simulink model "Quadcopter_State_model_Arduino"  (R2023b)
settings: Solver=VariableStepAuto  StartTime=0.0  StopTime=inf  FixedStep=0.00001  MinStep=0.001  RelTol=1e-3
model workspace (MAT data in the model file):
  DesiredPitchRoll : sugfis (value not decoded)
  DesiredThrust : sugfis (value not decoded)
  DesiredYaw : sugfis (value not decoded)
  Desired_Pitch = 0
  Desired_Roll = 0
  Desired_Yaw = 0
  Desired_Z_Velocity = -3
  FuzzyMotorspeed : sugfis (value not decoded)
values from neighbouring files (symbols this model uses):
  g = 9.81    [Quadcopter_Constants.m]
  Ixx = 0.0294838    [Quadcopter_Constants.m]
  Iyy = 0.0294838    [Quadcopter_Constants.m]
  Izz = 0.058967624    [Quadcopter_Constants.m]
  Jr = (6e-5)*1.358    (= 8.148e-05)    [Quadcopter_Constants.m]
  kd = 1    [Quadcopter_Constants.m]
  kd_phi = 1    [Quadcopter_Constants.m]
  kd_theta = 1    [Quadcopter_Constants.m]
  kf = 1    [Quadcopter_Constants.m]
  ki = 1    [Quadcopter_Constants.m]
  ki_phi = 1    [Quadcopter_Constants.m]
  ki_theta = 1    [Quadcopter_Constants.m]
  km = 4.74157e-9    (= 4.74157e-09)    [Quadcopter_Constants.m]
  kp = 1    [Quadcopter_Constants.m]
  kp_phi = 1    [Quadcopter_Constants.m]
  kp_theta = 1    [Quadcopter_Constants.m]
  kr = (0.1)*1.358    (= 0.1358)    [Quadcopter_Constants.m]
  kt = (0.1)*1.358    (= 0.1358)    [Quadcopter_Constants.m]
  l = 0.254    [Quadcopter_Constants.m]
  m = 0.914    [Quadcopter_Constants.m]
  sample_freq = 1000    [Quadcopter_Constants.m]
undefined symbols (not defined in the file or in its folder): LF
libraries: fuzblock x18, instrumentseriallib x12, simulink_extras x6, vrlib x4, instrumentlib x3, etargetslib x1, slpidlib x1, simulink x1
(part 5 of 5)

== system Quadcopter_State_model_Arduino/PID Simulation/Sensors/Sampling ==
  X_State : Inport
  Memory : Memory
  Square Wave Generator Enable : SignalGenerator  WaveForm=square  Frequency=sample_freq  Units=rad/sec
  Switch : Switch  Criteria=u2 > Threshold  SaturateOnIntegerOverflow=off  InputSameDT=off
  X_State Sensor : Outport
  wires:
  Switch/1 -> Memory/1
  Memory/1 -> X_State Sensor/1, Switch/3
  Square Wave Generator Enable/1 -> Switch/2
  X_State/1 -> Switch/1

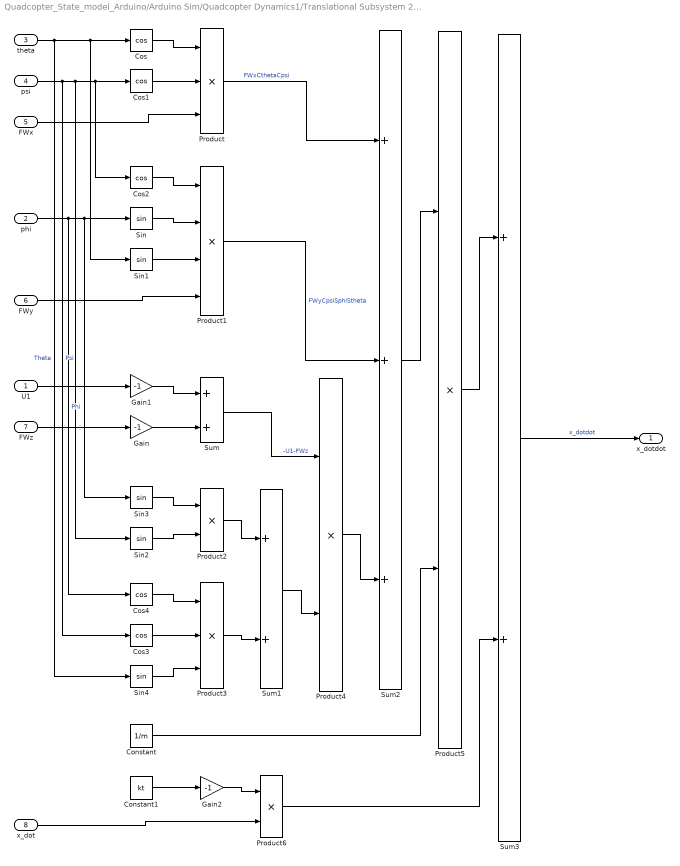
== system Quadcopter_State_model_Arduino/Arduino Sim/Quadcopter Dynamics1/Translational Subsystem 2.0/x_dotdot ==
  U1 : Inport
  phi : Inport  Port=2
  theta : Inport  Port=3
  psi : Inport  Port=4
  FWx : Inport  Port=5
  FWy : Inport  Port=6
  FWz : Inport  Port=7
  x_dot : Inport  Port=8
  Constant : Constant  Value=1/m
  Constant1 : Constant  Value=kt
  Cos{,1..4} (5 alike) : Trigonometry  Operator=cos
  Gain : Gain  Gain=-1
  Gain1 : Gain  Gain=-1
  Gain2 : Gain  Gain=-1
  Product : Product  Inputs=3
  Product1 : Product  Inputs=4
  Product{2,4..6} (4 alike) : Product
  Product3 : Product  Inputs=3
  Sin{,1..4} (5 alike) : Trigonometry
  Sum : Sum
  Sum1 : Sum
  Sum2 : Sum  Inputs=+++
  Sum3 : Sum
  x_dotdot : Outport
  wires:
  FWy/1 -> Product1/4
  x_dot/1 -> Product6/2
  U1/1 -> Gain1/1
  phi/1 -> Cos4/1, Sin3/1, Sin/1  "Phi"
  Cos1/1 -> Product/2
  FWx/1 -> Product/3
  psi/1 -> Cos3/1, Sin2/1, Cos2/1, Cos1/1  "Psi"
  Cos3/1 -> Product3/2
  Cos4/1 -> Product3/1
  Sin/1 -> Product1/2
  Product2/1 -> Sum1/1
  Gain1/1 -> Sum/1
  Sin4/1 -> Product3/3
  Product/1 -> Sum2/1  "FWxCthetaCpsi"
  Constant1/1 -> Gain2/1
  Product6/1 -> Sum3/2
  Sum3/1 -> x_dotdot/1  "x_dotdot"
  Cos/1 -> Product/1
  Gain2/1 -> Product6/1
  Constant/1 -> Product5/2
  Sin2/1 -> Product2/2
  Gain/1 -> Sum/2
  Product3/1 -> Sum1/2
  Sin3/1 -> Product2/1
  Product1/1 -> Sum2/2  "FWyCpsiSphiStheta"
  theta/1 -> Sin4/1, Sin1/1, Cos/1  "Theta"
  Sum2/1 -> Product5/1
  Sin1/1 -> Product1/3
  Cos2/1 -> Product1/1
  Product5/1 -> Sum3/1
  Sum/1 -> Product4/1  "-U1-FWz"
  FWz/1 -> Gain/1
  Sum1/1 -> Product4/2
  Product4/1 -> Sum2/3

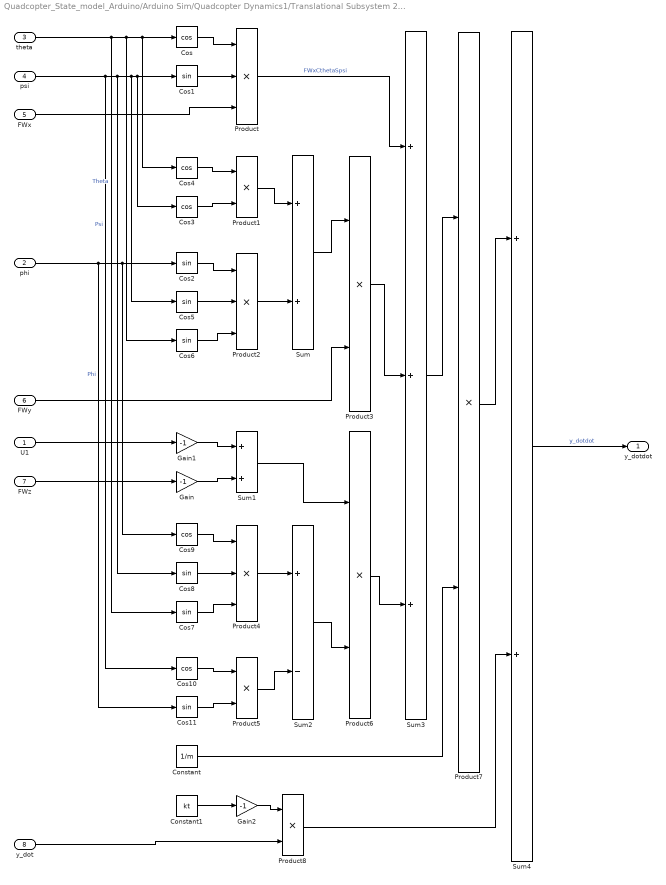
== system Quadcopter_State_model_Arduino/Arduino Sim/Quadcopter Dynamics1/Translational Subsystem 2.0/y_dotdot ==
  U1 : Inport
  phi : Inport  Port=2
  theta : Inport  Port=3
  psi : Inport  Port=4
  FWx : Inport  Port=5
  FWy : Inport  Port=6
  FWz : Inport  Port=7
  y_dot : Inport  Port=8
  Constant : Constant  Value=1/m
  Constant1 : Constant  Value=kt
  Cos{,3..4,9..10} (5 alike) : Trigonometry  Operator=cos
  Cos{1..2,5..8,11} (7 alike) : Trigonometry
  Gain : Gain  Gain=-1
  Gain1 : Gain  Gain=-1
  Gain2 : Gain  Gain=-1
  Product : Product  Inputs=3
  Product{1,3,5..8} (6 alike) : Product
  Product2 : Product  Inputs=3
  Product4 : Product  Inputs=3
  Sum : Sum
  Sum1 : Sum
  Sum2 : Sum  Inputs=+-
  Sum3 : Sum  Inputs=+++
  Sum4 : Sum
  y_dotdot : Outport
  wires:
  Product8/1 -> Sum4/2
  Product4/1 -> Sum2/1
  Gain/1 -> Sum1/2
  Sum2/1 -> Product6/2
  Product2/1 -> Sum/2
  Constant1/1 -> Gain2/1
  Cos2/1 -> Product2/1
  theta/1 -> Cos7/1, Cos6/1, Cos4/1, Cos/1  "Theta"
  psi/1 -> Cos10/1, Cos8/1, Cos5/1, Cos3/1, Cos1/1  "Psi"
  phi/1 -> Cos11/1, Cos9/1, Cos2/1  "Phi"
  Cos8/1 -> Product4/2
  Cos10/1 -> Product5/1
  y_dot/1 -> Product8/2
  FWy/1 -> Product3/2
  Cos1/1 -> Product/2
  Sum/1 -> Product3/1
  Cos5/1 -> Product2/2
  Gain2/1 -> Product8/1
  Sum4/1 -> y_dotdot/1  "y_dotdot"
  Product5/1 -> Sum2/2
  Cos3/1 -> Product1/2
  Product7/1 -> Sum4/1
  Gain1/1 -> Sum1/1
  FWx/1 -> Product/3
  Sum1/1 -> Product6/1
  Product3/1 -> Sum3/2
  Product6/1 -> Sum3/3
  Sum3/1 -> Product7/1
  Cos/1 -> Product/1
  Product/1 -> Sum3/1  "FWxCthetaSpsi"
  Cos6/1 -> Product2/3
  Cos7/1 -> Product4/3
  Cos4/1 -> Product1/1
  Cos9/1 -> Product4/1
  Cos11/1 -> Product5/2
  Product1/1 -> Sum/1
  U1/1 -> Gain1/1
  FWz/1 -> Gain/1
  Constant/1 -> Product7/2

== system Quadcopter_State_model_Arduino/Arduino Sim/Quadcopter Dynamics1/Translational Subsystem 2.0/z_dodot ==
  U1 : Inport
  phi : Inport  Port=2
  theta : Inport  Port=3
  FWx : Inport  Port=4
  FWy : Inport  Port=5
  FWz : Inport  Port=6
  z_dot : Inport  Port=7
  Constant : Constant  Value=kt
  Constant1 : Constant  Value=g
  Cos2 : Trigonometry  Operator=cos
  Cos3 : Trigonometry
  Cos4 : Trigonometry
  Cos5 : Trigonometry  Operator=cos
  Cos6 : Trigonometry  Operator=cos
  Gain{,1..2,4} (4 alike) : Gain  Gain=-1
  Gain3 : Gain  Gain=1/m
  Product : Product
  Product1 : Product  Inputs=3
  Product2 : Product  Inputs=3
  Product3 : Product
  Sum : Sum
  Sum1 : Sum  Inputs=+++
  Sum2 : Sum  Inputs=+++
  z_dotdot : Outport
  wires:
  Product3/1 -> Sum2/3
  FWy/1 -> Product1/3
  theta/1 -> Cos6/1, Cos2/1, Cos3/1  "Theta"
  z_dot/1 -> Product3/2
  phi/1 -> Cos5/1, Cos4/1  "Phi"
  Cos5/1 -> Product2/2
  Product1/1 -> Sum1/2
  Product2/1 -> Sum1/3
  Cos4/1 -> Product1/2
  U1/1 -> Gain/1
  Gain/1 -> Sum/1
  Cos2/1 -> Product1/1
  Sum/1 -> Product2/1
  Cos3/1 -> Product/2
  Gain3/1 -> Sum2/2
  Gain2/1 -> Product3/1
  FWx/1 -> Gain4/1
  Sum1/1 -> Gain3/1
  FWz/1 -> Gain1/1
  Constant/1 -> Gain2/1
  Cos6/1 -> Product2/3
  Product/1 -> Sum1/1
  Gain1/1 -> Sum/2
  Constant1/1 -> Sum2/1
  Sum2/1 -> z_dotdot/1  "z_dotdot"
  Gain4/1 -> Product/1

== system Quadcopter_State_model_Arduino/Arduino Sim/Quadcopter Dynamics1/Translational Wind Engine/Projected Areas ==
  theta : Inport
  psi : Inport  Port=2
  phi : Inport  Port=3
  Abs{,1..5} (6 alike) : Abs  SaturateOnIntegerOverflow=off
  Product{,1..5} (6 alike) : Product
  Sin{,1,4..5,8..9} (6 alike) : Trigonometry
  Sin{2..3,6..7,10..11} (6 alike) : Trigonometry  Operator=cos
  Sum : Sum
  Sum1 : Sum
  Sum2 : Sum
  Ax : Outport
  Ay : Outport  Port=2
  Az : Outport  Port=3
  wires:
  theta/1 -> Sin10/1, Sin8/1, Sin2/1, Sin/1  "theta"
  Sin6/1 -> Product3/1
  Sin9/1 -> Product4/2
  Product2/1 -> Abs2/1
  Abs2/1 -> Sum1/1
  Abs3/1 -> Sum1/2
  Sin1/1 -> Product/2
  Sin8/1 -> Product4/1
  Sin10/1 -> Product5/1
  Sin7/1 -> Product3/2
  Sin4/1 -> Product2/1
  Sin5/1 -> Product2/2
  Sin/1 -> Product/1
  Product3/1 -> Abs3/1
  Sum/1 -> Ax/1  "Ax"
  Product/1 -> Abs/1
  Product5/1 -> Abs5/1
  psi/1 -> Sin7/1, Sin5/1, Sin3/1, Sin1/1  "psi"
  Sin11/1 -> Product5/2
  Product1/1 -> Abs1/1
  Abs5/1 -> Sum2/2
  Abs4/1 -> Sum2/1
  Product4/1 -> Abs4/1
  Abs1/1 -> Sum/2
  Sin2/1 -> Product1/1
  Abs/1 -> Sum/1
  Sin3/1 -> Product1/2
  Sum1/1 -> Ay/1  "Ay"
  Sum2/1 -> Az/1  "Az"
  phi/1 -> Sin11/1, Sin9/1, Sin6/1, Sin4/1  "phi"

== system Quadcopter_State_model_Arduino/Arduino Sim/Quadcopter Dynamics1/Translational Wind Engine/Wind Forces ==
  Ax : Inport
  Ay : Inport  Port=2
  Az : Inport  Port=3
  VWx : Inport  Port=4
  VWy : Inport  Port=5
  VWz : Inport  Port=6
  Constant : Constant  Value=0.613
  Constant1 : Constant  Value=0.613
  Constant2 : Constant  Value=kt
  Constant3 : Constant  Value=kt
  Constant4 : Constant  Value=0.613
  Constant5 : Constant  Value=kt
  Product : Product  Inputs=4
  Product1 : Product  Inputs=4
  Product2 : Product  Inputs=4
  Square : Math  Operator=square
  Square1 : Math  Operator=square
  Square2 : Math  Operator=square
  FWx : Outport
  FWy : Outport  Port=2
  FWz : Outport  Port=3
  wires:
  VWz/1 -> Square2/1
  Constant4/1 -> Product2/1
  Square2/1 -> Product2/4
  Constant2/1 -> Product/3
  Ax/1 -> Product/2
  Constant5/1 -> Product2/3
  Square/1 -> Product/4
  Az/1 -> Product2/2
  Constant/1 -> Product/1
  VWx/1 -> Square/1
  Constant3/1 -> Product1/3
  VWy/1 -> Square1/1
  Square1/1 -> Product1/4
  Ay/1 -> Product1/2
  Product2/1 -> FWz/1  "FWz"
  Constant1/1 -> Product1/1
  Product/1 -> FWx/1  "FWx"
  Product1/1 -> FWy/1  "FWy"

== system Quadcopter_State_model_Arduino/Arduino Sim/Quadcopter Dynamics1/Translational Wind Engine/Wind Generation ==
  Constant1 : Constant  Value=0
  Constant3 : Constant  Value=0
  Constant5 : Constant  Value=0
  Enable Wind X : Constant  Value=0
  Enable Wind Y : Constant  Value=0
  Enable Wind Z : Constant  Value=0
  Random Number : RandomNumber  SampleTime=0.1
  Random Number1 : RandomNumber  SampleTime=0.1
  Random Number2 : RandomNumber  SampleTime=0.1
  Switch : Switch  Criteria=u2 > Threshold  SaturateOnIntegerOverflow=off  InputSameDT=off
  Switch1 : Switch  Criteria=u2 > Threshold  SaturateOnIntegerOverflow=off  InputSameDT=off
  Switch2 : Switch  Criteria=u2 > Threshold  SaturateOnIntegerOverflow=off  InputSameDT=off
  VWx : Outport
  VWy : Outport  Port=2
  VWz : Outport  Port=3
  wires:
  Random Number/1 -> Switch/1  "X wind"
  Constant3/1 -> Switch/3
  Enable Wind X/1 -> Switch/2  "Enable"
  Switch/1 -> VWx/1
  Constant1/1 -> Switch1/3
  Enable Wind Y/1 -> Switch1/2  "Enable"
  Random Number1/1 -> Switch1/1  "Y wind"
  Constant5/1 -> Switch2/3
  Enable Wind Z/1 -> Switch2/2  "Enable"
  Random Number2/1 -> Switch2/1  "Z wind"
  Switch2/1 -> VWz/1
  Switch1/1 -> VWy/1

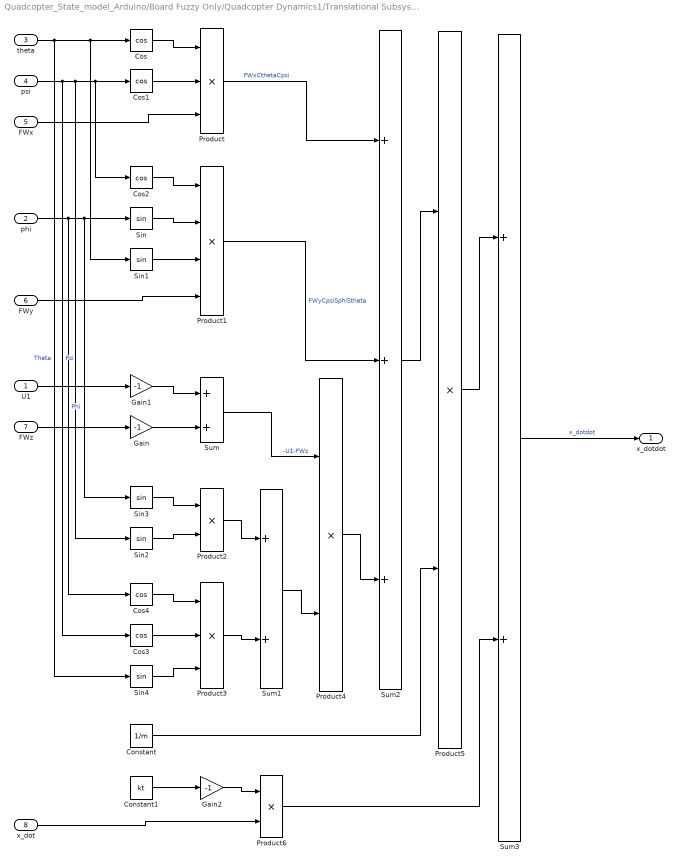
== system Quadcopter_State_model_Arduino/Board Fuzzy Only/Quadcopter Dynamics1/Translational Subsystem 2.0/x_dotdot ==
  U1 : Inport
  phi : Inport  Port=2
  theta : Inport  Port=3
  psi : Inport  Port=4
  FWx : Inport  Port=5
  FWy : Inport  Port=6
  FWz : Inport  Port=7
  x_dot : Inport  Port=8
  Constant : Constant  Value=1/m
  Constant1 : Constant  Value=kt
  Cos{,1..4} (5 alike) : Trigonometry  Operator=cos
  Gain : Gain  Gain=-1
  Gain1 : Gain  Gain=-1
  Gain2 : Gain  Gain=-1
  Product : Product  Inputs=3
  Product1 : Product  Inputs=4
  Product{2,4..6} (4 alike) : Product
  Product3 : Product  Inputs=3
  Sin{,1..4} (5 alike) : Trigonometry
  Sum : Sum
  Sum1 : Sum
  Sum2 : Sum  Inputs=+++
  Sum3 : Sum
  x_dotdot : Outport
  wires:
  FWy/1 -> Product1/4
  x_dot/1 -> Product6/2
  U1/1 -> Gain1/1
  phi/1 -> Cos4/1, Sin3/1, Sin/1  "Phi"
  Cos1/1 -> Product/2
  FWx/1 -> Product/3
  psi/1 -> Cos3/1, Sin2/1, Cos2/1, Cos1/1  "Psi"
  Cos3/1 -> Product3/2
  Cos4/1 -> Product3/1
  Sin/1 -> Product1/2
  Product2/1 -> Sum1/1
  Gain1/1 -> Sum/1
  Sin4/1 -> Product3/3
  Product/1 -> Sum2/1  "FWxCthetaCpsi"
  Constant1/1 -> Gain2/1
  Product6/1 -> Sum3/2
  Sum3/1 -> x_dotdot/1  "x_dotdot"
  Cos/1 -> Product/1
  Gain2/1 -> Product6/1
  Constant/1 -> Product5/2
  Sin2/1 -> Product2/2
  Gain/1 -> Sum/2
  Product3/1 -> Sum1/2
  Sin3/1 -> Product2/1
  Product1/1 -> Sum2/2  "FWyCpsiSphiStheta"
  theta/1 -> Sin4/1, Sin1/1, Cos/1  "Theta"
  Sum2/1 -> Product5/1
  Sin1/1 -> Product1/3
  Cos2/1 -> Product1/1
  Product5/1 -> Sum3/1
  Sum/1 -> Product4/1  "-U1-FWz"
  FWz/1 -> Gain/1
  Sum1/1 -> Product4/2
  Product4/1 -> Sum2/3

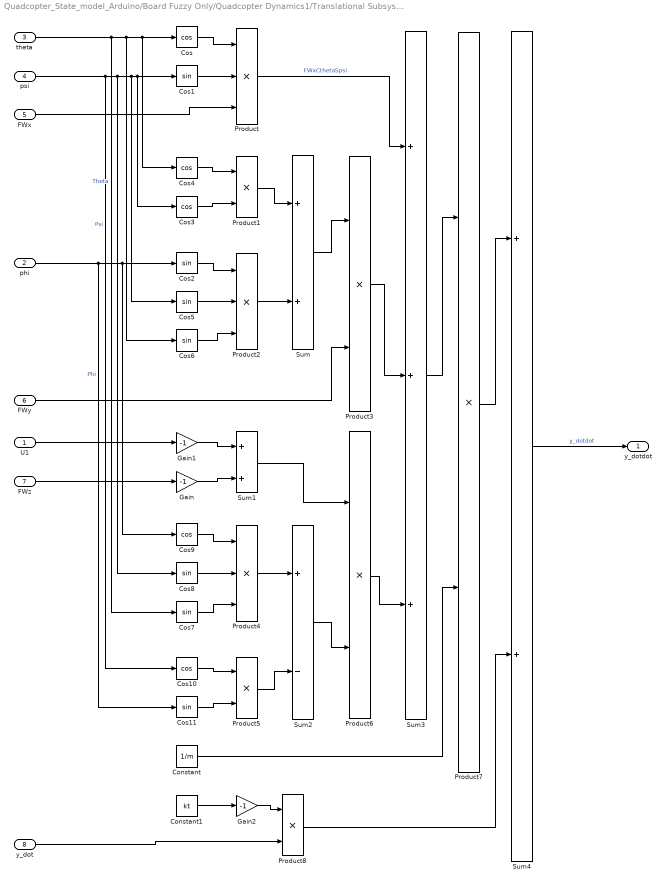
== system Quadcopter_State_model_Arduino/Board Fuzzy Only/Quadcopter Dynamics1/Translational Subsystem 2.0/y_dotdot ==
  U1 : Inport
  phi : Inport  Port=2
  theta : Inport  Port=3
  psi : Inport  Port=4
  FWx : Inport  Port=5
  FWy : Inport  Port=6
  FWz : Inport  Port=7
  y_dot : Inport  Port=8
  Constant : Constant  Value=1/m
  Constant1 : Constant  Value=kt
  Cos{,3..4,9..10} (5 alike) : Trigonometry  Operator=cos
  Cos{1..2,5..8,11} (7 alike) : Trigonometry
  Gain : Gain  Gain=-1
  Gain1 : Gain  Gain=-1
  Gain2 : Gain  Gain=-1
  Product : Product  Inputs=3
  Product{1,3,5..8} (6 alike) : Product
  Product2 : Product  Inputs=3
  Product4 : Product  Inputs=3
  Sum : Sum
  Sum1 : Sum
  Sum2 : Sum  Inputs=+-
  Sum3 : Sum  Inputs=+++
  Sum4 : Sum
  y_dotdot : Outport
  wires:
  Product8/1 -> Sum4/2
  Product4/1 -> Sum2/1
  Gain/1 -> Sum1/2
  Sum2/1 -> Product6/2
  Product2/1 -> Sum/2
  Constant1/1 -> Gain2/1
  Cos2/1 -> Product2/1
  theta/1 -> Cos7/1, Cos6/1, Cos4/1, Cos/1  "Theta"
  psi/1 -> Cos10/1, Cos8/1, Cos5/1, Cos3/1, Cos1/1  "Psi"
  phi/1 -> Cos11/1, Cos9/1, Cos2/1  "Phi"
  Cos8/1 -> Product4/2
  Cos10/1 -> Product5/1
  y_dot/1 -> Product8/2
  FWy/1 -> Product3/2
  Cos1/1 -> Product/2
  Sum/1 -> Product3/1
  Cos5/1 -> Product2/2
  Gain2/1 -> Product8/1
  Sum4/1 -> y_dotdot/1  "y_dotdot"
  Product5/1 -> Sum2/2
  Cos3/1 -> Product1/2
  Product7/1 -> Sum4/1
  Gain1/1 -> Sum1/1
  FWx/1 -> Product/3
  Sum1/1 -> Product6/1
  Product3/1 -> Sum3/2
  Product6/1 -> Sum3/3
  Sum3/1 -> Product7/1
  Cos/1 -> Product/1
  Product/1 -> Sum3/1  "FWxCthetaSpsi"
  Cos6/1 -> Product2/3
  Cos7/1 -> Product4/3
  Cos4/1 -> Product1/1
  Cos9/1 -> Product4/1
  Cos11/1 -> Product5/2
  Product1/1 -> Sum/1
  U1/1 -> Gain1/1
  FWz/1 -> Gain/1
  Constant/1 -> Product7/2

== system Quadcopter_State_model_Arduino/Board Fuzzy Only/Quadcopter Dynamics1/Translational Subsystem 2.0/z_dodot ==
  U1 : Inport
  phi : Inport  Port=2
  theta : Inport  Port=3
  FWx : Inport  Port=4
  FWy : Inport  Port=5
  FWz : Inport  Port=6
  z_dot : Inport  Port=7
  Constant : Constant  Value=kt
  Constant1 : Constant  Value=g
  Cos2 : Trigonometry  Operator=cos
  Cos3 : Trigonometry
  Cos4 : Trigonometry
  Cos5 : Trigonometry  Operator=cos
  Cos6 : Trigonometry  Operator=cos
  Gain{,1..2,4} (4 alike) : Gain  Gain=-1
  Gain3 : Gain  Gain=1/m
  Product : Product
  Product1 : Product  Inputs=3
  Product2 : Product  Inputs=3
  Product3 : Product
  Sum : Sum
  Sum1 : Sum  Inputs=+++
  Sum2 : Sum  Inputs=+++
  z_dotdot : Outport
  wires:
  Product3/1 -> Sum2/3
  FWy/1 -> Product1/3
  theta/1 -> Cos6/1, Cos2/1, Cos3/1  "Theta"
  z_dot/1 -> Product3/2
  phi/1 -> Cos5/1, Cos4/1  "Phi"
  Cos5/1 -> Product2/2
  Product1/1 -> Sum1/2
  Product2/1 -> Sum1/3
  Cos4/1 -> Product1/2
  U1/1 -> Gain/1
  Gain/1 -> Sum/1
  Cos2/1 -> Product1/1
  Sum/1 -> Product2/1
  Cos3/1 -> Product/2
  Gain3/1 -> Sum2/2
  Gain2/1 -> Product3/1
  FWx/1 -> Gain4/1
  Sum1/1 -> Gain3/1
  FWz/1 -> Gain1/1
  Constant/1 -> Gain2/1
  Cos6/1 -> Product2/3
  Product/1 -> Sum1/1
  Gain1/1 -> Sum/2
  Constant1/1 -> Sum2/1
  Sum2/1 -> z_dotdot/1  "z_dotdot"
  Gain4/1 -> Product/1

== system Quadcopter_State_model_Arduino/Board Fuzzy Only/Quadcopter Dynamics1/Translational Wind Engine/Projected Areas ==
  theta : Inport
  psi : Inport  Port=2
  phi : Inport  Port=3
  Abs{,1..5} (6 alike) : Abs  SaturateOnIntegerOverflow=off
  Product{,1..5} (6 alike) : Product
  Sin{,1,4..5,8..9} (6 alike) : Trigonometry
  Sin{2..3,6..7,10..11} (6 alike) : Trigonometry  Operator=cos
  Sum : Sum
  Sum1 : Sum
  Sum2 : Sum
  Ax : Outport
  Ay : Outport  Port=2
  Az : Outport  Port=3
  wires:
  theta/1 -> Sin10/1, Sin8/1, Sin2/1, Sin/1  "theta"
  Sin6/1 -> Product3/1
  Sin9/1 -> Product4/2
  Product2/1 -> Abs2/1
  Abs2/1 -> Sum1/1
  Abs3/1 -> Sum1/2
  Sin1/1 -> Product/2
  Sin8/1 -> Product4/1
  Sin10/1 -> Product5/1
  Sin7/1 -> Product3/2
  Sin4/1 -> Product2/1
  Sin5/1 -> Product2/2
  Sin/1 -> Product/1
  Product3/1 -> Abs3/1
  Sum/1 -> Ax/1  "Ax"
  Product/1 -> Abs/1
  Product5/1 -> Abs5/1
  psi/1 -> Sin7/1, Sin5/1, Sin3/1, Sin1/1  "psi"
  Sin11/1 -> Product5/2
  Product1/1 -> Abs1/1
  Abs5/1 -> Sum2/2
  Abs4/1 -> Sum2/1
  Product4/1 -> Abs4/1
  Abs1/1 -> Sum/2
  Sin2/1 -> Product1/1
  Abs/1 -> Sum/1
  Sin3/1 -> Product1/2
  Sum1/1 -> Ay/1  "Ay"
  Sum2/1 -> Az/1  "Az"
  phi/1 -> Sin11/1, Sin9/1, Sin6/1, Sin4/1  "phi"

== system Quadcopter_State_model_Arduino/Board Fuzzy Only/Quadcopter Dynamics1/Translational Wind Engine/Wind Forces ==
  Ax : Inport
  Ay : Inport  Port=2
  Az : Inport  Port=3
  VWx : Inport  Port=4
  VWy : Inport  Port=5
  VWz : Inport  Port=6
  Constant : Constant  Value=0.613
  Constant1 : Constant  Value=0.613
  Constant2 : Constant  Value=kt
  Constant3 : Constant  Value=kt
  Constant4 : Constant  Value=0.613
  Constant5 : Constant  Value=kt
  Product : Product  Inputs=4
  Product1 : Product  Inputs=4
  Product2 : Product  Inputs=4
  Square : Math  Operator=square
  Square1 : Math  Operator=square
  Square2 : Math  Operator=square
  FWx : Outport
  FWy : Outport  Port=2
  FWz : Outport  Port=3
  wires:
  VWz/1 -> Square2/1
  Constant4/1 -> Product2/1
  Square2/1 -> Product2/4
  Constant2/1 -> Product/3
  Ax/1 -> Product/2
  Constant5/1 -> Product2/3
  Square/1 -> Product/4
  Az/1 -> Product2/2
  Constant/1 -> Product/1
  VWx/1 -> Square/1
  Constant3/1 -> Product1/3
  VWy/1 -> Square1/1
  Square1/1 -> Product1/4
  Ay/1 -> Product1/2
  Product2/1 -> FWz/1  "FWz"
  Constant1/1 -> Product1/1
  Product/1 -> FWx/1  "FWx"
  Product1/1 -> FWy/1  "FWy"

== system Quadcopter_State_model_Arduino/Board Fuzzy Only/Quadcopter Dynamics1/Translational Wind Engine/Wind Generation ==
  Constant1 : Constant  Value=0
  Constant3 : Constant  Value=0
  Constant5 : Constant  Value=0
  Enable Wind X : Constant  Value=0
  Enable Wind Y : Constant  Value=0
  Enable Wind Z : Constant  Value=0
  Random Number : RandomNumber  SampleTime=0.1
  Random Number1 : RandomNumber  SampleTime=0.1
  Random Number2 : RandomNumber  SampleTime=0.1
  Switch : Switch  Criteria=u2 > Threshold  SaturateOnIntegerOverflow=off  InputSameDT=off
  Switch1 : Switch  Criteria=u2 > Threshold  SaturateOnIntegerOverflow=off  InputSameDT=off
  Switch2 : Switch  Criteria=u2 > Threshold  SaturateOnIntegerOverflow=off  InputSameDT=off
  VWx : Outport
  VWy : Outport  Port=2
  VWz : Outport  Port=3
  wires:
  Random Number/1 -> Switch/1  "X wind"
  Constant3/1 -> Switch/3
  Enable Wind X/1 -> Switch/2  "Enable"
  Switch/1 -> VWx/1
  Constant1/1 -> Switch1/3
  Enable Wind Y/1 -> Switch1/2  "Enable"
  Random Number1/1 -> Switch1/1  "Y wind"
  Constant5/1 -> Switch2/3
  Enable Wind Z/1 -> Switch2/2  "Enable"
  Random Number2/1 -> Switch2/1  "Z wind"
  Switch2/1 -> VWz/1
  Switch1/1 -> VWy/1

== system Quadcopter_State_model_Arduino/Fuzzy Simulation/Quadcopter Dynamics1/Translational Subsystem 2.0/x_dotdot ==
  U1 : Inport
  phi : Inport  Port=2
  theta : Inport  Port=3
  psi : Inport  Port=4
  FWx : Inport  Port=5
  FWy : Inport  Port=6
  FWz : Inport  Port=7
  x_dot : Inport  Port=8
  Constant : Constant  Value=1/m
  Constant1 : Constant  Value=kt
  Cos{,1..4} (5 alike) : Trigonometry  Operator=cos
  Gain : Gain  Gain=-1
  Gain1 : Gain  Gain=-1
  Gain2 : Gain  Gain=-1
  Product : Product  Inputs=3
  Product1 : Product  Inputs=4
  Product{2,4..6} (4 alike) : Product
  Product3 : Product  Inputs=3
  Sin{,1..4} (5 alike) : Trigonometry
  Sum : Sum
  Sum1 : Sum
  Sum2 : Sum  Inputs=+++
  Sum3 : Sum
  x_dotdot : Outport
  wires:
  FWy/1 -> Product1/4
  x_dot/1 -> Product6/2
  U1/1 -> Gain1/1
  phi/1 -> Cos4/1, Sin3/1, Sin/1  "Phi"
  Cos1/1 -> Product/2
  FWx/1 -> Product/3
  psi/1 -> Cos3/1, Sin2/1, Cos2/1, Cos1/1  "Psi"
  Cos3/1 -> Product3/2
  Cos4/1 -> Product3/1
  Sin/1 -> Product1/2
  Product2/1 -> Sum1/1
  Gain1/1 -> Sum/1
  Sin4/1 -> Product3/3
  Product/1 -> Sum2/1  "FWxCthetaCpsi"
  Constant1/1 -> Gain2/1
  Product6/1 -> Sum3/2
  Sum3/1 -> x_dotdot/1  "x_dotdot"
  Cos/1 -> Product/1
  Gain2/1 -> Product6/1
  Constant/1 -> Product5/2
  Sin2/1 -> Product2/2
  Gain/1 -> Sum/2
  Product3/1 -> Sum1/2
  Sin3/1 -> Product2/1
  Product1/1 -> Sum2/2  "FWyCpsiSphiStheta"
  theta/1 -> Sin4/1, Sin1/1, Cos/1  "Theta"
  Sum2/1 -> Product5/1
  Sin1/1 -> Product1/3
  Cos2/1 -> Product1/1
  Product5/1 -> Sum3/1
  Sum/1 -> Product4/1  "-U1-FWz"
  FWz/1 -> Gain/1
  Sum1/1 -> Product4/2
  Product4/1 -> Sum2/3

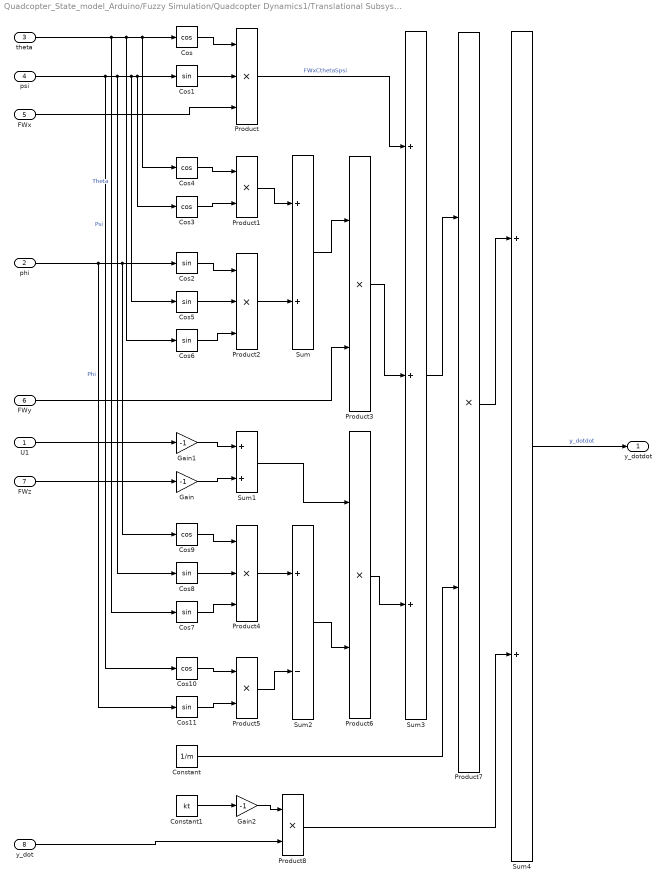
== system Quadcopter_State_model_Arduino/Fuzzy Simulation/Quadcopter Dynamics1/Translational Subsystem 2.0/y_dotdot ==
  U1 : Inport
  phi : Inport  Port=2
  theta : Inport  Port=3
  psi : Inport  Port=4
  FWx : Inport  Port=5
  FWy : Inport  Port=6
  FWz : Inport  Port=7
  y_dot : Inport  Port=8
  Constant : Constant  Value=1/m
  Constant1 : Constant  Value=kt
  Cos{,3..4,9..10} (5 alike) : Trigonometry  Operator=cos
  Cos{1..2,5..8,11} (7 alike) : Trigonometry
  Gain : Gain  Gain=-1
  Gain1 : Gain  Gain=-1
  Gain2 : Gain  Gain=-1
  Product : Product  Inputs=3
  Product{1,3,5..8} (6 alike) : Product
  Product2 : Product  Inputs=3
  Product4 : Product  Inputs=3
  Sum : Sum
  Sum1 : Sum
  Sum2 : Sum  Inputs=+-
  Sum3 : Sum  Inputs=+++
  Sum4 : Sum
  y_dotdot : Outport
  wires:
  Product8/1 -> Sum4/2
  Product4/1 -> Sum2/1
  Gain/1 -> Sum1/2
  Sum2/1 -> Product6/2
  Product2/1 -> Sum/2
  Constant1/1 -> Gain2/1
  Cos2/1 -> Product2/1
  theta/1 -> Cos7/1, Cos6/1, Cos4/1, Cos/1  "Theta"
  psi/1 -> Cos10/1, Cos8/1, Cos5/1, Cos3/1, Cos1/1  "Psi"
  phi/1 -> Cos11/1, Cos9/1, Cos2/1  "Phi"
  Cos8/1 -> Product4/2
  Cos10/1 -> Product5/1
  y_dot/1 -> Product8/2
  FWy/1 -> Product3/2
  Cos1/1 -> Product/2
  Sum/1 -> Product3/1
  Cos5/1 -> Product2/2
  Gain2/1 -> Product8/1
  Sum4/1 -> y_dotdot/1  "y_dotdot"
  Product5/1 -> Sum2/2
  Cos3/1 -> Product1/2
  Product7/1 -> Sum4/1
  Gain1/1 -> Sum1/1
  FWx/1 -> Product/3
  Sum1/1 -> Product6/1
  Product3/1 -> Sum3/2
  Product6/1 -> Sum3/3
  Sum3/1 -> Product7/1
  Cos/1 -> Product/1
  Product/1 -> Sum3/1  "FWxCthetaSpsi"
  Cos6/1 -> Product2/3
  Cos7/1 -> Product4/3
  Cos4/1 -> Product1/1
  Cos9/1 -> Product4/1
  Cos11/1 -> Product5/2
  Product1/1 -> Sum/1
  U1/1 -> Gain1/1
  FWz/1 -> Gain/1
  Constant/1 -> Product7/2

== system Quadcopter_State_model_Arduino/Fuzzy Simulation/Quadcopter Dynamics1/Translational Subsystem 2.0/z_dodot ==
  U1 : Inport
  phi : Inport  Port=2
  theta : Inport  Port=3
  FWx : Inport  Port=4
  FWy : Inport  Port=5
  FWz : Inport  Port=6
  z_dot : Inport  Port=7
  Constant : Constant  Value=kt
  Constant1 : Constant  Value=g
  Cos2 : Trigonometry  Operator=cos
  Cos3 : Trigonometry
  Cos4 : Trigonometry
  Cos5 : Trigonometry  Operator=cos
  Cos6 : Trigonometry  Operator=cos
  Gain{,1..2,4} (4 alike) : Gain  Gain=-1
  Gain3 : Gain  Gain=1/m
  Product : Product
  Product1 : Product  Inputs=3
  Product2 : Product  Inputs=3
  Product3 : Product
  Sum : Sum
  Sum1 : Sum  Inputs=+++
  Sum2 : Sum  Inputs=+++
  z_dotdot : Outport
  wires:
  Product3/1 -> Sum2/3
  FWy/1 -> Product1/3
  theta/1 -> Cos6/1, Cos2/1, Cos3/1  "Theta"
  z_dot/1 -> Product3/2
  phi/1 -> Cos5/1, Cos4/1  "Phi"
  Cos5/1 -> Product2/2
  Product1/1 -> Sum1/2
  Product2/1 -> Sum1/3
  Cos4/1 -> Product1/2
  U1/1 -> Gain/1
  Gain/1 -> Sum/1
  Cos2/1 -> Product1/1
  Sum/1 -> Product2/1
  Cos3/1 -> Product/2
  Gain3/1 -> Sum2/2
  Gain2/1 -> Product3/1
  FWx/1 -> Gain4/1
  Sum1/1 -> Gain3/1
  FWz/1 -> Gain1/1
  Constant/1 -> Gain2/1
  Cos6/1 -> Product2/3
  Product/1 -> Sum1/1
  Gain1/1 -> Sum/2
  Constant1/1 -> Sum2/1
  Sum2/1 -> z_dotdot/1  "z_dotdot"
  Gain4/1 -> Product/1

== system Quadcopter_State_model_Arduino/Fuzzy Simulation/Quadcopter Dynamics1/Translational Wind Engine/Projected Areas ==
  theta : Inport
  psi : Inport  Port=2
  phi : Inport  Port=3
  Abs{,1..5} (6 alike) : Abs  SaturateOnIntegerOverflow=off
  Product{,1..5} (6 alike) : Product
  Sin{,1,4..5,8..9} (6 alike) : Trigonometry
  Sin{2..3,6..7,10..11} (6 alike) : Trigonometry  Operator=cos
  Sum : Sum
  Sum1 : Sum
  Sum2 : Sum
  Ax : Outport
  Ay : Outport  Port=2
  Az : Outport  Port=3
  wires:
  theta/1 -> Sin10/1, Sin8/1, Sin2/1, Sin/1  "theta"
  Sin6/1 -> Product3/1
  Sin9/1 -> Product4/2
  Product2/1 -> Abs2/1
  Abs2/1 -> Sum1/1
  Abs3/1 -> Sum1/2
  Sin1/1 -> Product/2
  Sin8/1 -> Product4/1
  Sin10/1 -> Product5/1
  Sin7/1 -> Product3/2
  Sin4/1 -> Product2/1
  Sin5/1 -> Product2/2
  Sin/1 -> Product/1
  Product3/1 -> Abs3/1
  Sum/1 -> Ax/1  "Ax"
  Product/1 -> Abs/1
  Product5/1 -> Abs5/1
  psi/1 -> Sin7/1, Sin5/1, Sin3/1, Sin1/1  "psi"
  Sin11/1 -> Product5/2
  Product1/1 -> Abs1/1
  Abs5/1 -> Sum2/2
  Abs4/1 -> Sum2/1
  Product4/1 -> Abs4/1
  Abs1/1 -> Sum/2
  Sin2/1 -> Product1/1
  Abs/1 -> Sum/1
  Sin3/1 -> Product1/2
  Sum1/1 -> Ay/1  "Ay"
  Sum2/1 -> Az/1  "Az"
  phi/1 -> Sin11/1, Sin9/1, Sin6/1, Sin4/1  "phi"

== system Quadcopter_State_model_Arduino/Fuzzy Simulation/Quadcopter Dynamics1/Translational Wind Engine/Wind Forces ==
  Ax : Inport
  Ay : Inport  Port=2
  Az : Inport  Port=3
  VWx : Inport  Port=4
  VWy : Inport  Port=5
  VWz : Inport  Port=6
  Constant : Constant  Value=0.613
  Constant1 : Constant  Value=0.613
  Constant2 : Constant  Value=kt
  Constant3 : Constant  Value=kt
  Constant4 : Constant  Value=0.613
  Constant5 : Constant  Value=kt
  Product : Product  Inputs=4
  Product1 : Product  Inputs=4
  Product2 : Product  Inputs=4
  Square : Math  Operator=square
  Square1 : Math  Operator=square
  Square2 : Math  Operator=square
  FWx : Outport
  FWy : Outport  Port=2
  FWz : Outport  Port=3
  wires:
  VWz/1 -> Square2/1
  Constant4/1 -> Product2/1
  Square2/1 -> Product2/4
  Constant2/1 -> Product/3
  Ax/1 -> Product/2
  Constant5/1 -> Product2/3
  Square/1 -> Product/4
  Az/1 -> Product2/2
  Constant/1 -> Product/1
  VWx/1 -> Square/1
  Constant3/1 -> Product1/3
  VWy/1 -> Square1/1
  Square1/1 -> Product1/4
  Ay/1 -> Product1/2
  Product2/1 -> FWz/1  "FWz"
  Constant1/1 -> Product1/1
  Product/1 -> FWx/1  "FWx"
  Product1/1 -> FWy/1  "FWy"

== system Quadcopter_State_model_Arduino/Fuzzy Simulation/Quadcopter Dynamics1/Translational Wind Engine/Wind Generation ==
  Constant1 : Constant  Value=0
  Constant3 : Constant  Value=0
  Constant5 : Constant  Value=0
  Enable Wind X : Constant  Value=0
  Enable Wind Y : Constant  Value=0
  Enable Wind Z : Constant  Value=0
  Random Number : RandomNumber  SampleTime=0.1
  Random Number1 : RandomNumber  SampleTime=0.1
  Random Number2 : RandomNumber  SampleTime=0.1
  Switch : Switch  Criteria=u2 > Threshold  SaturateOnIntegerOverflow=off  InputSameDT=off
  Switch1 : Switch  Criteria=u2 > Threshold  SaturateOnIntegerOverflow=off  InputSameDT=off
  Switch2 : Switch  Criteria=u2 > Threshold  SaturateOnIntegerOverflow=off  InputSameDT=off
  VWx : Outport
  VWy : Outport  Port=2
  VWz : Outport  Port=3
  wires:
  Random Number/1 -> Switch/1  "X wind"
  Constant3/1 -> Switch/3
  Enable Wind X/1 -> Switch/2  "Enable"
  Switch/1 -> VWx/1
  Constant1/1 -> Switch1/3
  Enable Wind Y/1 -> Switch1/2  "Enable"
  Random Number1/1 -> Switch1/1  "Y wind"
  Constant5/1 -> Switch2/3
  Enable Wind Z/1 -> Switch2/2  "Enable"
  Random Number2/1 -> Switch2/1  "Z wind"
  Switch2/1 -> VWz/1
  Switch1/1 -> VWy/1

== system Quadcopter_State_model_Arduino/PID Simulation/Controller_Subsystem/ /Attitude Controller ==
  e_phi : Inport
  e_theta : Inport  Port=2
  Derivative : Derivative
  Derivative1 : Derivative
  Gain : Gain  Gain=kd_phi
  Gain1 : Gain  Gain=kp_phi
  Gain2 : Gain  Gain=ki_phi
  Gain3 : Gain  Gain=kd_theta
  Gain4 : Gain  Gain=kp_theta
  Gain5 : Gain  Gain=ki_theta
  Integrator : Integrator
  Integrator1 : Integrator
  Sum1 : Sum  Inputs=+++
  Sum2 : Sum  Inputs=+++
  U2 : Outport
  U3 : Outport  Port=2
  wires:
  Gain/1 -> Derivative/1
  Sum1/1 -> U2/1  "U2"
  Gain1/1 -> Sum1/2
  e_phi/1 -> Gain2/1, Gain1/1, Gain/1
  Gain2/1 -> Integrator/1
  Gain5/1 -> Integrator1/1
  e_theta/1 -> Gain5/1, Gain4/1, Gain3/1
  Gain4/1 -> Sum2/2
  Sum2/1 -> U3/1  "U3"
  Gain3/1 -> Derivative1/1
  Derivative/1 -> Sum1/1
  Derivative1/1 -> Sum2/1
  Integrator/1 -> Sum1/3
  Integrator1/1 -> Sum2/3

== system Quadcopter_State_model_Arduino/PID Simulation/Controller_Subsystem/ /World to Body Conversion ==
  note: X_transformed = x*cos(psi) - y*sin(psi)
      | Y_transformed = x*sin(psi) + y*cos(psi)
  note: Stole this from MIT
  e_y : Inport
  e_x : Inport  Port=2
  psi : Inport  Port=3
  Gain : Gain  Gain=-1
  Gain1 : Gain  Gain=.024
  Gain2 : Gain  Gain=.024
  Product{,1..3} (4 alike) : Product
  Saturation2 : Saturate  UpperLimit=0.3  LowerLimit=-0.3
  Saturation3 : Saturate  UpperLimit=0.3  LowerLimit=-0.3
  Scope : Scope  NumInputPorts=4
  Sum : Sum
  Sum1 : Sum
  cos : Trigonometry  Operator=cos
  sin : Trigonometry
  phi_d : Outport
  theta_d : Outport  Port=2
  wires:
  psi/1 -> cos/1, sin/1
  sin/1 -> Product2/1, Gain/1
  cos/1 -> Product3/1, Product/1
  Product/1 -> Sum/1
  Product1/1 -> Sum/2
  Sum/1 -> Gain1/1, Scope/3  "e_x_transform"
  Product3/1 -> Sum1/2
  Product2/1 -> Sum1/1
  Sum1/1 -> Gain2/1, Scope/4  "e_y_transform"
  e_x/1 -> Product2/2, Product/2, Scope/1
  Gain/1 -> Product1/1
  e_y/1 -> Product3/2, Product1/2, Scope/2
  Gain1/1 -> Saturation2/1
  Gain2/1 -> Saturation3/1
  Saturation2/1 -> theta_d/1
  Saturation3/1 -> phi_d/1

== system Quadcopter_State_model_Arduino/PID Simulation/Quadcopter Dynamics/Translational Subsystem 2.0/x_dotdot ==
  U1 : Inport
  phi : Inport  Port=2
  theta : Inport  Port=3
  psi : Inport  Port=4
  FWx : Inport  Port=5
  FWy : Inport  Port=6
  FWz : Inport  Port=7
  x_dot : Inport  Port=8
  Constant : Constant  Value=1/m
  Constant1 : Constant  Value=kt
  Cos{,1..4} (5 alike) : Trigonometry  Operator=cos
  Gain : Gain  Gain=-1
  Gain1 : Gain  Gain=-1
  Gain2 : Gain  Gain=-1
  Product : Product  Inputs=3
  Product1 : Product  Inputs=4
  Product{2,4..6} (4 alike) : Product
  Product3 : Product  Inputs=3
  Sin{,1..4} (5 alike) : Trigonometry
  Sum : Sum
  Sum1 : Sum
  Sum2 : Sum  Inputs=+++
  Sum3 : Sum
  x_dotdot : Outport
  wires:
  FWy/1 -> Product1/4
  x_dot/1 -> Product6/2
  U1/1 -> Gain1/1
  phi/1 -> Cos4/1, Sin3/1, Sin/1  "Phi"
  Cos1/1 -> Product/2
  FWx/1 -> Product/3
  psi/1 -> Cos3/1, Sin2/1, Cos2/1, Cos1/1  "Psi"
  Cos3/1 -> Product3/2
  Cos4/1 -> Product3/1
  Sin/1 -> Product1/2
  Product2/1 -> Sum1/1
  Gain1/1 -> Sum/1
  Sin4/1 -> Product3/3
  Product/1 -> Sum2/1  "FWxCthetaCpsi"
  Constant1/1 -> Gain2/1
  Product6/1 -> Sum3/2
  Sum3/1 -> x_dotdot/1  "x_dotdot"
  Cos/1 -> Product/1
  Gain2/1 -> Product6/1
  Constant/1 -> Product5/2
  Sin2/1 -> Product2/2
  Gain/1 -> Sum/2
  Product3/1 -> Sum1/2
  Sin3/1 -> Product2/1
  Product1/1 -> Sum2/2  "FWyCpsiSphiStheta"
  theta/1 -> Sin4/1, Sin1/1, Cos/1  "Theta"
  Sum2/1 -> Product5/1
  Sin1/1 -> Product1/3
  Cos2/1 -> Product1/1
  Product5/1 -> Sum3/1
  Sum/1 -> Product4/1  "-U1-FWz"
  FWz/1 -> Gain/1
  Sum1/1 -> Product4/2
  Product4/1 -> Sum2/3

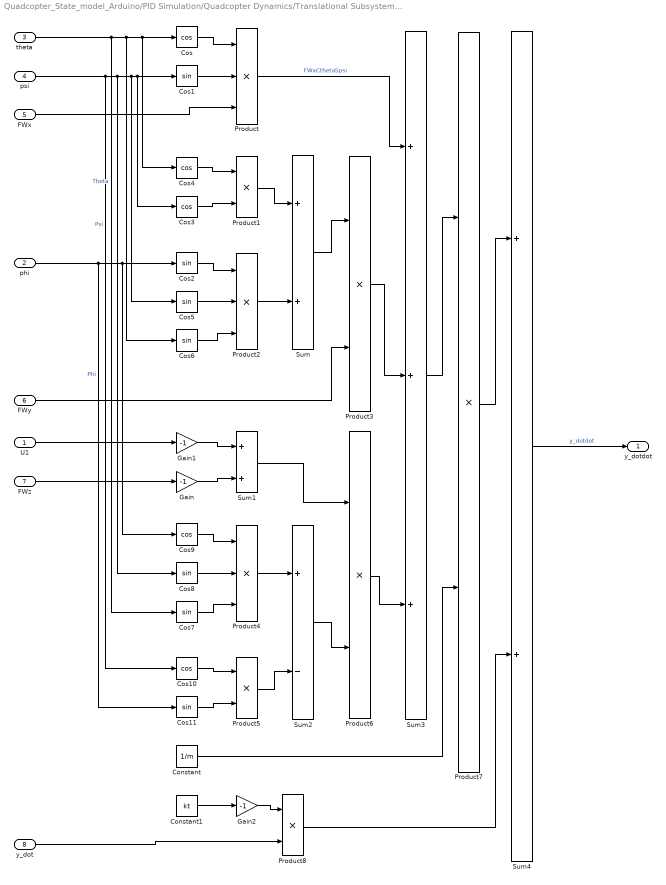
== system Quadcopter_State_model_Arduino/PID Simulation/Quadcopter Dynamics/Translational Subsystem 2.0/y_dotdot ==
  U1 : Inport
  phi : Inport  Port=2
  theta : Inport  Port=3
  psi : Inport  Port=4
  FWx : Inport  Port=5
  FWy : Inport  Port=6
  FWz : Inport  Port=7
  y_dot : Inport  Port=8
  Constant : Constant  Value=1/m
  Constant1 : Constant  Value=kt
  Cos{,3..4,9..10} (5 alike) : Trigonometry  Operator=cos
  Cos{1..2,5..8,11} (7 alike) : Trigonometry
  Gain : Gain  Gain=-1
  Gain1 : Gain  Gain=-1
  Gain2 : Gain  Gain=-1
  Product : Product  Inputs=3
  Product{1,3,5..8} (6 alike) : Product
  Product2 : Product  Inputs=3
  Product4 : Product  Inputs=3
  Sum : Sum
  Sum1 : Sum
  Sum2 : Sum  Inputs=+-
  Sum3 : Sum  Inputs=+++
  Sum4 : Sum
  y_dotdot : Outport
  wires:
  Product8/1 -> Sum4/2
  Product4/1 -> Sum2/1
  Gain/1 -> Sum1/2
  Sum2/1 -> Product6/2
  Product2/1 -> Sum/2
  Constant1/1 -> Gain2/1
  Cos2/1 -> Product2/1
  theta/1 -> Cos7/1, Cos6/1, Cos4/1, Cos/1  "Theta"
  psi/1 -> Cos10/1, Cos8/1, Cos5/1, Cos3/1, Cos1/1  "Psi"
  phi/1 -> Cos11/1, Cos9/1, Cos2/1  "Phi"
  Cos8/1 -> Product4/2
  Cos10/1 -> Product5/1
  y_dot/1 -> Product8/2
  FWy/1 -> Product3/2
  Cos1/1 -> Product/2
  Sum/1 -> Product3/1
  Cos5/1 -> Product2/2
  Gain2/1 -> Product8/1
  Sum4/1 -> y_dotdot/1  "y_dotdot"
  Product5/1 -> Sum2/2
  Cos3/1 -> Product1/2
  Product7/1 -> Sum4/1
  Gain1/1 -> Sum1/1
  FWx/1 -> Product/3
  Sum1/1 -> Product6/1
  Product3/1 -> Sum3/2
  Product6/1 -> Sum3/3
  Sum3/1 -> Product7/1
  Cos/1 -> Product/1
  Product/1 -> Sum3/1  "FWxCthetaSpsi"
  Cos6/1 -> Product2/3
  Cos7/1 -> Product4/3
  Cos4/1 -> Product1/1
  Cos9/1 -> Product4/1
  Cos11/1 -> Product5/2
  Product1/1 -> Sum/1
  U1/1 -> Gain1/1
  FWz/1 -> Gain/1
  Constant/1 -> Product7/2

== system Quadcopter_State_model_Arduino/PID Simulation/Quadcopter Dynamics/Translational Subsystem 2.0/z_dodot ==
  U1 : Inport
  phi : Inport  Port=2
  theta : Inport  Port=3
  FWx : Inport  Port=4
  FWy : Inport  Port=5
  FWz : Inport  Port=6
  z_dot : Inport  Port=7
  Constant : Constant  Value=kt
  Constant1 : Constant  Value=g
  Cos2 : Trigonometry  Operator=cos
  Cos3 : Trigonometry
  Cos4 : Trigonometry
  Cos5 : Trigonometry  Operator=cos
  Cos6 : Trigonometry  Operator=cos
  Gain{,1..2,4} (4 alike) : Gain  Gain=-1
  Gain3 : Gain  Gain=1/m
  Product : Product
  Product1 : Product  Inputs=3
  Product2 : Product  Inputs=3
  Product3 : Product
  Sum : Sum
  Sum1 : Sum  Inputs=+++
  Sum2 : Sum  Inputs=+++
  z_dotdot : Outport
  wires:
  Product3/1 -> Sum2/3
  FWy/1 -> Product1/3
  theta/1 -> Cos6/1, Cos2/1, Cos3/1  "Theta"
  z_dot/1 -> Product3/2
  phi/1 -> Cos5/1, Cos4/1  "Phi"
  Cos5/1 -> Product2/2
  Product1/1 -> Sum1/2
  Product2/1 -> Sum1/3
  Cos4/1 -> Product1/2
  U1/1 -> Gain/1
  Gain/1 -> Sum/1
  Cos2/1 -> Product1/1
  Sum/1 -> Product2/1
  Cos3/1 -> Product/2
  Gain3/1 -> Sum2/2
  Gain2/1 -> Product3/1
  FWx/1 -> Gain4/1
  Sum1/1 -> Gain3/1
  FWz/1 -> Gain1/1
  Constant/1 -> Gain2/1
  Cos6/1 -> Product2/3
  Product/1 -> Sum1/1
  Gain1/1 -> Sum/2
  Constant1/1 -> Sum2/1
  Sum2/1 -> z_dotdot/1  "z_dotdot"
  Gain4/1 -> Product/1

== system Quadcopter_State_model_Arduino/PID Simulation/Quadcopter Dynamics/Translational Wind Engine/Projected Areas ==
  theta : Inport
  psi : Inport  Port=2
  phi : Inport  Port=3
  Abs{,1..5} (6 alike) : Abs  SaturateOnIntegerOverflow=off
  Product{,1..5} (6 alike) : Product
  Sin{,1,4..5,8..9} (6 alike) : Trigonometry
  Sin{2..3,6..7,10..11} (6 alike) : Trigonometry  Operator=cos
  Sum : Sum
  Sum1 : Sum
  Sum2 : Sum
  Ax : Outport
  Ay : Outport  Port=2
  Az : Outport  Port=3
  wires:
  theta/1 -> Sin10/1, Sin8/1, Sin2/1, Sin/1  "theta"
  Sin6/1 -> Product3/1
  Sin9/1 -> Product4/2
  Product2/1 -> Abs2/1
  Abs2/1 -> Sum1/1
  Abs3/1 -> Sum1/2
  Sin1/1 -> Product/2
  Sin8/1 -> Product4/1
  Sin10/1 -> Product5/1
  Sin7/1 -> Product3/2
  Sin4/1 -> Product2/1
  Sin5/1 -> Product2/2
  Sin/1 -> Product/1
  Product3/1 -> Abs3/1
  Sum/1 -> Ax/1  "Ax"
  Product/1 -> Abs/1
  Product5/1 -> Abs5/1
  psi/1 -> Sin7/1, Sin5/1, Sin3/1, Sin1/1  "psi"
  Sin11/1 -> Product5/2
  Product1/1 -> Abs1/1
  Abs5/1 -> Sum2/2
  Abs4/1 -> Sum2/1
  Product4/1 -> Abs4/1
  Abs1/1 -> Sum/2
  Sin2/1 -> Product1/1
  Abs/1 -> Sum/1
  Sin3/1 -> Product1/2
  Sum1/1 -> Ay/1  "Ay"
  Sum2/1 -> Az/1  "Az"
  phi/1 -> Sin11/1, Sin9/1, Sin6/1, Sin4/1  "phi"

== system Quadcopter_State_model_Arduino/PID Simulation/Quadcopter Dynamics/Translational Wind Engine/Wind Forces ==
  Ax : Inport
  Ay : Inport  Port=2
  Az : Inport  Port=3
  VWx : Inport  Port=4
  VWy : Inport  Port=5
  VWz : Inport  Port=6
  Constant : Constant  Value=0.613
  Constant1 : Constant  Value=0.613
  Constant2 : Constant  Value=kt
  Constant3 : Constant  Value=kt
  Constant4 : Constant  Value=0.613
  Constant5 : Constant  Value=kt
  Product : Product  Inputs=4
  Product1 : Product  Inputs=4
  Product2 : Product  Inputs=4
  Square : Math  Operator=square
  Square1 : Math  Operator=square
  Square2 : Math  Operator=square
  FWx : Outport
  FWy : Outport  Port=2
  FWz : Outport  Port=3
  wires:
  VWz/1 -> Square2/1
  Constant4/1 -> Product2/1
  Square2/1 -> Product2/4
  Constant2/1 -> Product/3
  Ax/1 -> Product/2
  Constant5/1 -> Product2/3
  Square/1 -> Product/4
  Az/1 -> Product2/2
  Constant/1 -> Product/1
  VWx/1 -> Square/1
  Constant3/1 -> Product1/3
  VWy/1 -> Square1/1
  Square1/1 -> Product1/4
  Ay/1 -> Product1/2
  Product2/1 -> FWz/1  "FWz"
  Constant1/1 -> Product1/1
  Product/1 -> FWx/1  "FWx"
  Product1/1 -> FWy/1  "FWy"

== system Quadcopter_State_model_Arduino/PID Simulation/Quadcopter Dynamics/Translational Wind Engine/Wind Generation ==
  Constant1 : Constant  Value=0
  Constant3 : Constant  Value=0
  Constant5 : Constant  Value=0
  Enable Wind X : Constant  Value=0
  Enable Wind Y : Constant  Value=0
  Enable Wind Z : Constant  Value=0
  Random Number : RandomNumber  SampleTime=0.1
  Random Number1 : RandomNumber  SampleTime=0.1
  Random Number2 : RandomNumber  SampleTime=0.1
  Switch : Switch  Criteria=u2 > Threshold  SaturateOnIntegerOverflow=off  InputSameDT=off
  Switch1 : Switch  Criteria=u2 > Threshold  SaturateOnIntegerOverflow=off  InputSameDT=off
  Switch2 : Switch  Criteria=u2 > Threshold  SaturateOnIntegerOverflow=off  InputSameDT=off
  VWx : Outport
  VWy : Outport  Port=2
  VWz : Outport  Port=3
  wires:
  Random Number/1 -> Switch/1  "X wind"
  Constant3/1 -> Switch/3
  Enable Wind X/1 -> Switch/2  "Enable"
  Switch/1 -> VWx/1
  Constant1/1 -> Switch1/3
  Enable Wind Y/1 -> Switch1/2  "Enable"
  Random Number1/1 -> Switch1/1  "Y wind"
  Constant5/1 -> Switch2/3
  Enable Wind Z/1 -> Switch2/2  "Enable"
  Random Number2/1 -> Switch2/1  "Z wind"
  Switch2/1 -> VWz/1
  Switch1/1 -> VWy/1

== matlab function Quadcopter_State_model_Arduino/Fuzzy Simulation/Arduino Communication/MATLAB Function ==
  data: m input; m1o output; m2o output; m3o output; m4o output
function [m1o,m2o,m3o,m4o] = fcn(m)

    m1o = m(1);
    m2o = m(2);
    m3o = m(3);
    m4o = m(4);

end

== matlab function Quadcopter_State_model_Arduino/Arduino Sim/Arduino Communication/MATLAB Function ==
  data: m input; m1o output; m2o output; m3o output; m4o output
function [m1o,m2o,m3o,m4o] = fcn(m)

    m1o = m(1);
    m2o = m(2);
    m3o = m(3);
    m4o = m(4);

end

== matlab function Quadcopter_State_model_Arduino/Arduino Sim/Visualization/Inertal to body frame ==
  data: phi input; R output size=[3 3]; theta input; psi input
function R = fcn(phi, theta, psi)

Rx = [1 0 0; 0 cos(phi) -sin(phi); 0 sin(phi) cos(phi)];
Ry = [cos(theta) 0 sin(theta); 0 1 0; -sin(theta) 0 cos(theta)];
Rz = [cos(psi) -sin(psi) 0; sin(psi) cos(psi) 0; 0 0 1];

R = Rx*Ry*Rz;

== matlab function Quadcopter_State_model_Arduino/PID Simulation/Visualization/Inertal to body frame ==
  data: phi input; R output size=[3 3]; theta input; psi input
function R = fcn(phi, theta, psi)

Rx = [1 0 0; 0 cos(phi) -sin(phi); 0 sin(phi) cos(phi)];
Ry = [cos(theta) 0 sin(theta); 0 1 0; -sin(theta) 0 cos(theta)];
Rz = [cos(psi) -sin(psi) 0; sin(psi) cos(psi) 0; 0 0 1];

R = Rx*Ry*Rz;
